simulink model "frekvens"  (Simulink 5.0)
settings: Solver=ode45  SolverMode=SingleTasking  StartTime=-1  StopTime=120.0  RelTol=1e-3
undefined symbols (not defined in the file): D, fref, J, K, PDC, Pe, Pref, R, wnom
settings Model: Creator=ielolof  LastModifiedBy=ielolof  ExtModeAutoUpdateStatusClock=off  LimitDataPoints=off  BooleanDataType=off

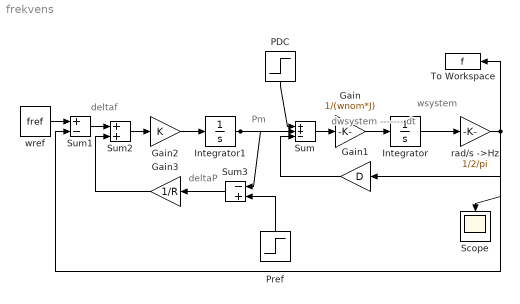
== system frekvens ==
  note: Pm
  note: deltaf
  note: deltaP
  note: dwsystem
      | -------
      | dt
  note: wsystem
  Gain : Gain  Gain=1/(wnom*J)  SaturateOnIntegerOverflow=on
  Gain1 : Gain  Orientation=left  Gain=D  SaturateOnIntegerOverflow=on
  Gain2 : Gain  Gain=K  SaturateOnIntegerOverflow=on
  Gain3 : Gain  Orientation=left  Gain=1/R  SaturateOnIntegerOverflow=on
  Integrator : Integrator  InitialCondition=100*pi
  Integrator1 : Integrator  InitialCondition=Pe-PDC
  PDC : Step  Orientation=down  Time=0  Before=PDC  After=0  SampleTime=0
  Pref : Step  Orientation=up  Time=1000  Before=Pref  After=Pref+PDC  SampleTime=0
  Scope : Scope
      settings: Orientation=down  TickLabels=on  TimeRange=140  YMin=49.5  YMax=50  DataFormat=Array
  Sum : Sum  Inputs=++-  SaturateOnIntegerOverflow=on  InputSameDT=on
  Sum1 : Sum  Inputs=+-  SaturateOnIntegerOverflow=on  InputSameDT=on
  Sum2 : Sum  SaturateOnIntegerOverflow=on  InputSameDT=on
  Sum3 : Sum  Orientation=left  Inputs=-+  SaturateOnIntegerOverflow=on  InputSameDT=on
  To Workspace : ToWorkspace  VariableName=f  SampleTime=-1  SaveFormat=Array
  rad/s ->Hz : Gain  Gain=1/2/pi  SaturateOnIntegerOverflow=on
  wref : Constant  Value=fref
  wires:
  Sum/1 -> Gain/1
  Gain/1 -> Integrator/1
  Gain1/1 -> Sum/3
  PDC/1 -> Sum/1
  Sum1/1 -> Sum2/1
  Integrator1/1 -> Sum/2, Sum3/1
  Sum3/1 -> Gain3/1
  Gain3/1 -> Sum2/2
  Sum2/1 -> Gain2/1
  Gain2/1 -> Integrator1/1
  wref/1 -> Sum1/1
  Pref/1 -> Sum3/2
  rad/s ->Hz/1 -> Scope/1, To Workspace/1, Gain1/1, Sum1/2
  Integrator/1 -> rad/s ->Hz/1
